simulink model "controller_sdfp_host"  (Simulink 7.8)
settings: Solver=ode3  StartTime=0.0  StopTime=1  RelTol=1e-3
values from neighbouring files (symbols this model uses):
  delay_shift1 = -k_preint    (= 0)    [one_bit_control.m]
  delay_shift2 = -k_preint    (= 0)    [one_bit_control.m]
  delay_shift3 = -k_preint    (= 0)    [one_bit_control.m]
  fixpt_adder_in_bitwidth = w    (= 24)    [one_bit_control.m]    (also in reconstruction_filter_setup.m)
  fixpt_adder_in_position = d    (= 16)    [one_bit_control.m]    (also in reconstruction_filter_setup.m)
  fixpt_adder_out_bitwidth = w    (= 24)    [one_bit_control.m]    (also in reconstruction_filter_setup.m)
  fixpt_adder_out_position = d    (= 16)    [one_bit_control.m]    (also in reconstruction_filter_setup.m)
  fixpt_gain_bitwidth = w    (= 24)    [one_bit_control.m]    (also in reconstruction_filter_setup.m)
  fixpt_gain_position = d    (= 16)    [one_bit_control.m]    (also in reconstruction_filter_setup.m)
  k = 2^k_bitshift    (= 0.000244140625)    [one_bit_control.m]
  p0 = 1326*T^3*k^-3    [one_bit_control.m]
  p1 = 9397*T^2*k^-2    [one_bit_control.m]
  p2 = 262.3*T*k^-1    [one_bit_control.m]
  p3 = 16.65    [one_bit_control.m]
  postint_gain1 = k_postint    (= -12)    [one_bit_control.m]
  postint_gain2 = k_postint    (= -12)    [one_bit_control.m]
  postint_gain3 = k_postint    (= -12)    [one_bit_control.m]
  preint_gain1 = k_preint    (= 0)    [one_bit_control.m]
  preint_gain2 = k_preint    (= 0)    [one_bit_control.m]
  preint_gain3 = k_preint    (= 0)    [one_bit_control.m]
  q0 = 0*T^3*k^-3    [one_bit_control.m]
  q1 = 400.8*T^2*k^-2    [one_bit_control.m]
  q2 = 33.2*T*k^-1    [one_bit_control.m]
  T = ts    [one_bit_control.m]
  ts = 1/Fs    [one_bit_control.m]
libraries: simulink x4, commnoisgen2 x1, cstblocks x1
(part 2 of 2)

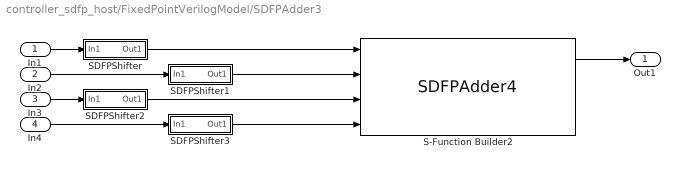
== system controller_sdfp_host/FixedPointVerilogModel/SDFPAdder3 ==
  In1 : Inport
  In2 : Inport  Port=2
  In3 : Inport  Port=3
  In4 : Inport  Port=4
  S-Function Builder2 : S-Function  InitFcn=try, set_param(gcb,'FunctionName','SDFPAdder4'), end  FunctionName=SDFPAdder4  Parameters=uint32(in_bitwidth),uint32(in_fp_position),uint32(out_bitwidth),uint32(out_fp_position)  SFunctionModules=SDFPAdder4_wrapper  WizardData=DataTag25  EnableBusSupport=off  mask(S-Function Builder){}
      mask help: The S-Function Builder block creates a wrapper C-MEX S-function from your supplied C code with multiple input ports, output ports, and a variable number of scalar, vector, or matrix parameters. The input and output ports can propagate Simulink built-in data types, fixed-point datatypes, complex, frame, 1-D, and 2-D signals. This block also supports discrete and continuous states of type real. You can optionally have the block generate a TLC file to be used with Real-Time Workshop for code generation.
      mask init: same as controller_sdfp_host/FixedPointVerilogModel/FloatForScope1/S-Function Builder
      settings: CopyFcn=set_param(gcbh,'LinkStatus','none')  PreSaveFcn=try, set_param(gcb,'FunctionName','SDFPAdder4'), end  OpenFcn=sfunctionwizard(gcbh)
      mask Display: plot(val(:,1),val(:,2)),disp(sys)port_label('input',1,'in0')port_label('input',2,'in1')port_label('input',3,'in2')port_label('input',4,'in3')port_label('output',1,'adder_out')port_label('output',2,'DBG_in01')port_label('output',3,'DBG_in012')
  SDFPShifter : Subsystem  mask{shift_amount=in1_shift}
      mask init:
      | if(shift_amount > 0)
      |     dispval=sprintf('<< %d',shift_amount);
      | else
      |     dispval=sprintf('>> %d',-shift_amount);
      | end
      mask Display: disp(dispval);
  SDFPShifter1 : Subsystem  mask{shift_amount=in2_shift}
      mask init:
      | if(shift_amount > 0)
      |     dispval=sprintf('<< %d',shift_amount);
      | else
      |     dispval=sprintf('>> %d',-shift_amount);
      | end
      mask Display: disp(dispval);
  SDFPShifter2 : Subsystem  mask{shift_amount=in3_shift}
      mask init:
      | if(shift_amount > 0)
      |     dispval=sprintf('<< %d',shift_amount);
      | else
      |     dispval=sprintf('>> %d',-shift_amount);
      | end
      mask Display: disp(dispval);
  SDFPShifter3 : Subsystem  mask{shift_amount=in4_shift}
      mask init:
      | if(shift_amount > 0)
      |     dispval=sprintf('<< %d',shift_amount);
      | else
      |     dispval=sprintf('>> %d',-shift_amount);
      | end
      mask Display: disp(dispval);
  Out1 : Outport
  wires:
  In1/1 -> SDFPShifter/1(In1)
  In2/1 -> SDFPShifter1/1(In1)
  In3/1 -> SDFPShifter2/1(In1)
  In4/1 -> SDFPShifter3/1(In1)
  S-Function Builder2/1 -> Out1/1
  SDFPShifter/1(Out1) -> S-Function Builder2/1
  SDFPShifter1/1(Out1) -> S-Function Builder2/2
  SDFPShifter2/1(Out1) -> S-Function Builder2/3
  SDFPShifter3/1(Out1) -> S-Function Builder2/4

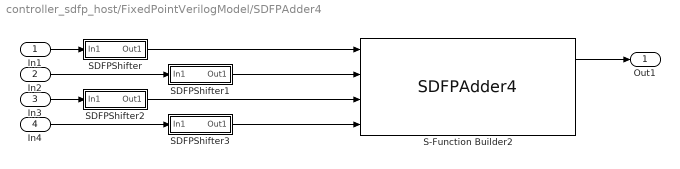
== system controller_sdfp_host/FixedPointVerilogModel/SDFPAdder4 ==
  In1 : Inport
  In2 : Inport  Port=2
  In3 : Inport  Port=3
  In4 : Inport  Port=4
  S-Function Builder2 : S-Function  InitFcn=try, set_param(gcb,'FunctionName','SDFPAdder4'), end  FunctionName=SDFPAdder4  Parameters=uint32(in_bitwidth),uint32(in_fp_position),uint32(out_bitwidth),uint32(out_fp_position)  SFunctionModules=SDFPAdder4_wrapper  WizardData=DataTag30  EnableBusSupport=off  mask(S-Function Builder){}
      mask help: The S-Function Builder block creates a wrapper C-MEX S-function from your supplied C code with multiple input ports, output ports, and a variable number of scalar, vector, or matrix parameters. The input and output ports can propagate Simulink built-in data types, fixed-point datatypes, complex, frame, 1-D, and 2-D signals. This block also supports discrete and continuous states of type real. You can optionally have the block generate a TLC file to be used with Real-Time Workshop for code generation.
      mask init: same as controller_sdfp_host/FixedPointVerilogModel/FloatForScope1/S-Function Builder
      settings: CopyFcn=set_param(gcbh,'LinkStatus','none')  PreSaveFcn=try, set_param(gcb,'FunctionName','SDFPAdder4'), end  OpenFcn=sfunctionwizard(gcbh)
      mask Display: plot(val(:,1),val(:,2)),disp(sys)port_label('input',1,'in0')port_label('input',2,'in1')port_label('input',3,'in2')port_label('input',4,'in3')port_label('output',1,'adder_out')port_label('output',2,'DBG_in01')port_label('output',3,'DBG_in012')
  SDFPShifter : Subsystem  mask{shift_amount=in1_shift}
      mask init:
      | if(shift_amount > 0)
      |     dispval=sprintf('<< %d',shift_amount);
      | else
      |     dispval=sprintf('>> %d',-shift_amount);
      | end
      mask Display: disp(dispval);
  SDFPShifter1 : Subsystem  mask{shift_amount=in2_shift}
      mask init:
      | if(shift_amount > 0)
      |     dispval=sprintf('<< %d',shift_amount);
      | else
      |     dispval=sprintf('>> %d',-shift_amount);
      | end
      mask Display: disp(dispval);
  SDFPShifter2 : Subsystem  mask{shift_amount=in3_shift}
      mask init:
      | if(shift_amount > 0)
      |     dispval=sprintf('<< %d',shift_amount);
      | else
      |     dispval=sprintf('>> %d',-shift_amount);
      | end
      mask Display: disp(dispval);
  SDFPShifter3 : Subsystem  mask{shift_amount=in4_shift}
      mask init:
      | if(shift_amount > 0)
      |     dispval=sprintf('<< %d',shift_amount);
      | else
      |     dispval=sprintf('>> %d',-shift_amount);
      | end
      mask Display: disp(dispval);
  Out1 : Outport
  wires:
  SDFPShifter3/1(Out1) -> S-Function Builder2/4
  SDFPShifter2/1(Out1) -> S-Function Builder2/3
  SDFPShifter1/1(Out1) -> S-Function Builder2/2
  SDFPShifter/1(Out1) -> S-Function Builder2/1
  S-Function Builder2/1 -> Out1/1
  In4/1 -> SDFPShifter3/1(In1)
  In3/1 -> SDFPShifter2/1(In1)
  In2/1 -> SDFPShifter1/1(In1)
  In1/1 -> SDFPShifter/1(In1)

== system controller_sdfp_host/FixedPointVerilogModel/ts_and_k_gain1 ==
  In1 : Inport
  S-Function Builder3 : S-Function  InitFcn=try, set_param(gcb,'FunctionName','SDFPShifter'), end  FunctionName=SDFPShifter  Parameters=int32(shift_amount)  SFunctionModules=SDFPShifter_wrapper  WizardData=DataTag35  EnableBusSupport=off  mask(S-Function Builder){}
      mask help: The S-Function Builder block creates a wrapper C-MEX S-function from your supplied C code with multiple input ports, output ports, and a variable number of scalar, vector, or matrix parameters. The input and output ports can propagate Simulink built-in data types, fixed-point datatypes, complex, frame, 1-D, and 2-D signals. This block also supports discrete and continuous states of type real. You can optionally have the block generate a TLC file to be used with Real-Time Workshop for code generation.
      mask init: same as controller_sdfp_host/FixedPointVerilogModel/FloatForScope1/S-Function Builder
      settings: CopyFcn=set_param(gcbh,'LinkStatus','none')  PreSaveFcn=try, set_param(gcb,'FunctionName','SDFPShifter'), end  OpenFcn=sfunctionwizard(gcbh)
      mask Display: plot(val(:,1),val(:,2)),disp(sys)port_label('input',1,'sg_in')port_label('output',1,'shifter_out')
  Out1 : Outport
  wires:
  In1/1 -> S-Function Builder3/1
  S-Function Builder3/1 -> Out1/1

== system controller_sdfp_host/FixedPointVerilogModel/ts_and_k_gain2 ==
  In1 : Inport
  S-Function Builder3 : S-Function  InitFcn=try, set_param(gcb,'FunctionName','SDFPShifter'), end  FunctionName=SDFPShifter  Parameters=int32(shift_amount)  SFunctionModules=SDFPShifter_wrapper  WizardData=DataTag36  EnableBusSupport=off  mask(S-Function Builder){}
      mask help: The S-Function Builder block creates a wrapper C-MEX S-function from your supplied C code with multiple input ports, output ports, and a variable number of scalar, vector, or matrix parameters. The input and output ports can propagate Simulink built-in data types, fixed-point datatypes, complex, frame, 1-D, and 2-D signals. This block also supports discrete and continuous states of type real. You can optionally have the block generate a TLC file to be used with Real-Time Workshop for code generation.
      mask init: same as controller_sdfp_host/FixedPointVerilogModel/FloatForScope1/S-Function Builder
      settings: CopyFcn=set_param(gcbh,'LinkStatus','none')  PreSaveFcn=try, set_param(gcb,'FunctionName','SDFPShifter'), end  OpenFcn=sfunctionwizard(gcbh)
      mask Display: plot(val(:,1),val(:,2)),disp(sys)port_label('input',1,'sg_in')port_label('output',1,'shifter_out')
  Out1 : Outport
  wires:
  S-Function Builder3/1 -> Out1/1
  In1/1 -> S-Function Builder3/1

== system controller_sdfp_host/FixedPointVerilogModel/ts_and_k_gain3 ==
  In1 : Inport
  S-Function Builder3 : S-Function  InitFcn=try, set_param(gcb,'FunctionName','SDFPShifter'), end  FunctionName=SDFPShifter  Parameters=int32(shift_amount)  SFunctionModules=SDFPShifter_wrapper  WizardData=DataTag37  EnableBusSupport=off  mask(S-Function Builder){}
      mask help: The S-Function Builder block creates a wrapper C-MEX S-function from your supplied C code with multiple input ports, output ports, and a variable number of scalar, vector, or matrix parameters. The input and output ports can propagate Simulink built-in data types, fixed-point datatypes, complex, frame, 1-D, and 2-D signals. This block also supports discrete and continuous states of type real. You can optionally have the block generate a TLC file to be used with Real-Time Workshop for code generation.
      mask init: same as controller_sdfp_host/FixedPointVerilogModel/FloatForScope1/S-Function Builder
      settings: CopyFcn=set_param(gcbh,'LinkStatus','none')  PreSaveFcn=try, set_param(gcb,'FunctionName','SDFPShifter'), end  OpenFcn=sfunctionwizard(gcbh)
      mask Display: plot(val(:,1),val(:,2)),disp(sys)port_label('input',1,'sg_in')port_label('output',1,'shifter_out')
  Out1 : Outport
  wires:
  In1/1 -> S-Function Builder3/1
  S-Function Builder3/1 -> Out1/1

== system controller_sdfp_host/FixedPointVerilogModel/ts_and_k_gain4 ==
  In1 : Inport
  S-Function Builder3 : S-Function  InitFcn=try, set_param(gcb,'FunctionName','SDFPShifter'), end  FunctionName=SDFPShifter  Parameters=int32(shift_amount)  SFunctionModules=SDFPShifter_wrapper  WizardData=DataTag38  EnableBusSupport=off  mask(S-Function Builder){}
      mask help: The S-Function Builder block creates a wrapper C-MEX S-function from your supplied C code with multiple input ports, output ports, and a variable number of scalar, vector, or matrix parameters. The input and output ports can propagate Simulink built-in data types, fixed-point datatypes, complex, frame, 1-D, and 2-D signals. This block also supports discrete and continuous states of type real. You can optionally have the block generate a TLC file to be used with Real-Time Workshop for code generation.
      mask init: same as controller_sdfp_host/FixedPointVerilogModel/FloatForScope1/S-Function Builder
      settings: CopyFcn=set_param(gcbh,'LinkStatus','none')  PreSaveFcn=try, set_param(gcb,'FunctionName','SDFPShifter'), end  OpenFcn=sfunctionwizard(gcbh)
      mask Display: plot(val(:,1),val(:,2)),disp(sys)port_label('input',1,'sg_in')port_label('output',1,'shifter_out')
  Out1 : Outport
  wires:
  In1/1 -> S-Function Builder3/1
  S-Function Builder3/1 -> Out1/1

== system controller_sdfp_host/FixedPointVerilogModel/ts_and_k_gain5 ==
  In1 : Inport
  S-Function Builder3 : S-Function  InitFcn=try, set_param(gcb,'FunctionName','SDFPShifter'), end  FunctionName=SDFPShifter  Parameters=int32(shift_amount)  SFunctionModules=SDFPShifter_wrapper  WizardData=DataTag39  EnableBusSupport=off  mask(S-Function Builder){}
      mask help: The S-Function Builder block creates a wrapper C-MEX S-function from your supplied C code with multiple input ports, output ports, and a variable number of scalar, vector, or matrix parameters. The input and output ports can propagate Simulink built-in data types, fixed-point datatypes, complex, frame, 1-D, and 2-D signals. This block also supports discrete and continuous states of type real. You can optionally have the block generate a TLC file to be used with Real-Time Workshop for code generation.
      mask init: same as controller_sdfp_host/FixedPointVerilogModel/FloatForScope1/S-Function Builder
      settings: CopyFcn=set_param(gcbh,'LinkStatus','none')  PreSaveFcn=try, set_param(gcb,'FunctionName','SDFPShifter'), end  OpenFcn=sfunctionwizard(gcbh)
      mask Display: plot(val(:,1),val(:,2)),disp(sys)port_label('input',1,'sg_in')port_label('output',1,'shifter_out')
  Out1 : Outport
  wires:
  In1/1 -> S-Function Builder3/1
  S-Function Builder3/1 -> Out1/1

== system controller_sdfp_host/FixedPointVerilogModel/ts_and_k_gain6 ==
  In1 : Inport
  S-Function Builder3 : S-Function  InitFcn=try, set_param(gcb,'FunctionName','SDFPShifter'), end  FunctionName=SDFPShifter  Parameters=int32(shift_amount)  SFunctionModules=SDFPShifter_wrapper  WizardData=DataTag40  EnableBusSupport=off  mask(S-Function Builder){}
      mask help: The S-Function Builder block creates a wrapper C-MEX S-function from your supplied C code with multiple input ports, output ports, and a variable number of scalar, vector, or matrix parameters. The input and output ports can propagate Simulink built-in data types, fixed-point datatypes, complex, frame, 1-D, and 2-D signals. This block also supports discrete and continuous states of type real. You can optionally have the block generate a TLC file to be used with Real-Time Workshop for code generation.
      mask init: same as controller_sdfp_host/FixedPointVerilogModel/FloatForScope1/S-Function Builder
      settings: CopyFcn=set_param(gcbh,'LinkStatus','none')  PreSaveFcn=try, set_param(gcb,'FunctionName','SDFPShifter'), end  OpenFcn=sfunctionwizard(gcbh)
      mask Display: plot(val(:,1),val(:,2)),disp(sys)port_label('input',1,'sg_in')port_label('output',1,'shifter_out')
  Out1 : Outport
  wires:
  S-Function Builder3/1 -> Out1/1
  In1/1 -> S-Function Builder3/1

== system controller_sdfp_host/SecondOrder Sigdel1/Compare to Zero ==
  In1 : Inport
  Compare To Zero : simulink/Logic and Bit Operations/Compare To Zero  relop=>=  OutDataTypeStr=uint8
  Constant : Constant
  Constant1 : Constant  Value=-1
  Switch : Switch  Threshold=0.5
  Out1 : Outport
  wires:
  Constant1/1 -> Switch/3
  Constant/1 -> Switch/1
  Compare To Zero/1 -> Switch/2
  In1/1 -> Compare To Zero/1
  Switch/1 -> Out1/1

== system controller_sdfp_host/SecondOrder Sigdel2/Compare to Zero ==
  In1 : Inport
  Compare To Zero : simulink/Logic and Bit Operations/Compare To Zero  relop=>=  OutDataTypeStr=uint8
  Constant : Constant
  Constant1 : Constant  Value=-1
  Switch : Switch  Threshold=0.5
  Out1 : Outport
  wires:
  Constant1/1 -> Switch/3
  Constant/1 -> Switch/1
  Compare To Zero/1 -> Switch/2
  In1/1 -> Compare To Zero/1
  Switch/1 -> Out1/1

== system controller_sdfp_host/SecondOrder Sigdel3/Compare to Zero ==
  In1 : Inport
  Compare To Zero : simulink/Logic and Bit Operations/Compare To Zero  relop=>=  OutDataTypeStr=uint8
  Constant : Constant
  Constant1 : Constant  Value=-1
  Switch : Switch  Threshold=0.5
  Out1 : Outport
  wires:
  Constant1/1 -> Switch/3
  Constant/1 -> Switch/1
  Compare To Zero/1 -> Switch/2
  In1/1 -> Compare To Zero/1
  Switch/1 -> Out1/1

== system controller_sdfp_host/FixedPointVerilogModel/SDFPAdder1/GM1Float ==
  In1 : Inport
  S-Function Builder : S-Function  InitFcn=try, set_param(gcb,'FunctionName','SDFPFromFixed'), end  FunctionName=SDFPFromFixed  Parameters=uint32(bitwidth),uint32(fp_position)  SFunctionModules=SDFPFromFixed_wrapper fpconv  WizardData=DataTag13  EnableBusSupport=off  mask(S-Function Builder){}
      mask help: The S-Function Builder block creates a wrapper C-MEX S-function from your supplied C code with multiple input ports, output ports, and a variable number of scalar, vector, or matrix parameters. The input and output ports can propagate Simulink built-in data types, fixed-point datatypes, complex, frame, 1-D, and 2-D signals. This block also supports discrete and continuous states of type real. You can optionally have the block generate a TLC file to be used with Real-Time Workshop for code generation.
      mask init: same as controller_sdfp_host/FixedPointVerilogModel/FloatForScope1/S-Function Builder
      settings: CopyFcn=set_param(gcbh,'LinkStatus','none')  PreSaveFcn=try, set_param(gcb,'FunctionName','SDFPFromFixed'), end  OpenFcn=sfunctionwizard(gcbh)
      mask Display: plot(val(:,1),val(:,2)),disp(sys)port_label('input',1,'fixed_in')port_label('output',1,'float_out')
  Out1 : Outport
  wires:
  In1/1 -> S-Function Builder/1
  S-Function Builder/1 -> Out1/1

== system controller_sdfp_host/FixedPointVerilogModel/SDFPAdder1/GM1Float1 ==
  In1 : Inport
  S-Function Builder : S-Function  InitFcn=try, set_param(gcb,'FunctionName','SDFPFromFixed'), end  FunctionName=SDFPFromFixed  Parameters=uint32(bitwidth),uint32(fp_position)  SFunctionModules=SDFPFromFixed_wrapper fpconv  WizardData=DataTag14  EnableBusSupport=off  mask(S-Function Builder){}
      mask help: The S-Function Builder block creates a wrapper C-MEX S-function from your supplied C code with multiple input ports, output ports, and a variable number of scalar, vector, or matrix parameters. The input and output ports can propagate Simulink built-in data types, fixed-point datatypes, complex, frame, 1-D, and 2-D signals. This block also supports discrete and continuous states of type real. You can optionally have the block generate a TLC file to be used with Real-Time Workshop for code generation.
      mask init: same as controller_sdfp_host/FixedPointVerilogModel/FloatForScope1/S-Function Builder
      settings: CopyFcn=set_param(gcbh,'LinkStatus','none')  PreSaveFcn=try, set_param(gcb,'FunctionName','SDFPFromFixed'), end  OpenFcn=sfunctionwizard(gcbh)
      mask Display: plot(val(:,1),val(:,2)),disp(sys)port_label('input',1,'fixed_in')port_label('output',1,'float_out')
  Out1 : Outport
  wires:
  In1/1 -> S-Function Builder/1
  S-Function Builder/1 -> Out1/1

== system controller_sdfp_host/FixedPointVerilogModel/SDFPAdder1/SDFPShifter ==
  In1 : Inport
  S-Function Builder3 : S-Function  InitFcn=try, set_param(gcb,'FunctionName','SDFPShifter'), end  FunctionName=SDFPShifter  Parameters=int32(shift_amount)  SFunctionModules=SDFPShifter_wrapper  WizardData=DataTag16  EnableBusSupport=off  mask(S-Function Builder){}
      mask help: The S-Function Builder block creates a wrapper C-MEX S-function from your supplied C code with multiple input ports, output ports, and a variable number of scalar, vector, or matrix parameters. The input and output ports can propagate Simulink built-in data types, fixed-point datatypes, complex, frame, 1-D, and 2-D signals. This block also supports discrete and continuous states of type real. You can optionally have the block generate a TLC file to be used with Real-Time Workshop for code generation.
      mask init: same as controller_sdfp_host/FixedPointVerilogModel/FloatForScope1/S-Function Builder
      settings: CopyFcn=set_param(gcbh,'LinkStatus','none')  PreSaveFcn=try, set_param(gcb,'FunctionName','SDFPShifter'), end  OpenFcn=sfunctionwizard(gcbh)
      mask Display: plot(val(:,1),val(:,2)),disp(sys)port_label('input',1,'sg_in')port_label('output',1,'shifter_out')
  Out1 : Outport
  wires:
  In1/1 -> S-Function Builder3/1
  S-Function Builder3/1 -> Out1/1

== system controller_sdfp_host/FixedPointVerilogModel/SDFPAdder1/SDFPShifter1 ==
  In1 : Inport
  S-Function Builder3 : S-Function  InitFcn=try, set_param(gcb,'FunctionName','SDFPShifter'), end  FunctionName=SDFPShifter  Parameters=int32(shift_amount)  SFunctionModules=SDFPShifter_wrapper  WizardData=DataTag17  EnableBusSupport=off  mask(S-Function Builder){}
      mask help: The S-Function Builder block creates a wrapper C-MEX S-function from your supplied C code with multiple input ports, output ports, and a variable number of scalar, vector, or matrix parameters. The input and output ports can propagate Simulink built-in data types, fixed-point datatypes, complex, frame, 1-D, and 2-D signals. This block also supports discrete and continuous states of type real. You can optionally have the block generate a TLC file to be used with Real-Time Workshop for code generation.
      mask init: same as controller_sdfp_host/FixedPointVerilogModel/FloatForScope1/S-Function Builder
      settings: CopyFcn=set_param(gcbh,'LinkStatus','none')  PreSaveFcn=try, set_param(gcb,'FunctionName','SDFPShifter'), end  OpenFcn=sfunctionwizard(gcbh)
      mask Display: plot(val(:,1),val(:,2)),disp(sys)port_label('input',1,'sg_in')port_label('output',1,'shifter_out')
  Out1 : Outport
  wires:
  S-Function Builder3/1 -> Out1/1
  In1/1 -> S-Function Builder3/1

== system controller_sdfp_host/FixedPointVerilogModel/SDFPAdder1/SDFPShifter2 ==
  In1 : Inport
  S-Function Builder3 : S-Function  InitFcn=try, set_param(gcb,'FunctionName','SDFPShifter'), end  FunctionName=SDFPShifter  Parameters=int32(shift_amount)  SFunctionModules=SDFPShifter_wrapper  WizardData=DataTag18  EnableBusSupport=off  mask(S-Function Builder){}
      mask help: The S-Function Builder block creates a wrapper C-MEX S-function from your supplied C code with multiple input ports, output ports, and a variable number of scalar, vector, or matrix parameters. The input and output ports can propagate Simulink built-in data types, fixed-point datatypes, complex, frame, 1-D, and 2-D signals. This block also supports discrete and continuous states of type real. You can optionally have the block generate a TLC file to be used with Real-Time Workshop for code generation.
      mask init: same as controller_sdfp_host/FixedPointVerilogModel/FloatForScope1/S-Function Builder
      settings: CopyFcn=set_param(gcbh,'LinkStatus','none')  PreSaveFcn=try, set_param(gcb,'FunctionName','SDFPShifter'), end  OpenFcn=sfunctionwizard(gcbh)
      mask Display: plot(val(:,1),val(:,2)),disp(sys)port_label('input',1,'sg_in')port_label('output',1,'shifter_out')
  Out1 : Outport
  wires:
  In1/1 -> S-Function Builder3/1
  S-Function Builder3/1 -> Out1/1

== system controller_sdfp_host/FixedPointVerilogModel/SDFPAdder1/SDFPShifter3 ==
  In1 : Inport
  S-Function Builder3 : S-Function  InitFcn=try, set_param(gcb,'FunctionName','SDFPShifter'), end  FunctionName=SDFPShifter  Parameters=int32(shift_amount)  SFunctionModules=SDFPShifter_wrapper  WizardData=DataTag19  EnableBusSupport=off  mask(S-Function Builder){}
      mask help: The S-Function Builder block creates a wrapper C-MEX S-function from your supplied C code with multiple input ports, output ports, and a variable number of scalar, vector, or matrix parameters. The input and output ports can propagate Simulink built-in data types, fixed-point datatypes, complex, frame, 1-D, and 2-D signals. This block also supports discrete and continuous states of type real. You can optionally have the block generate a TLC file to be used with Real-Time Workshop for code generation.
      mask init: same as controller_sdfp_host/FixedPointVerilogModel/FloatForScope1/S-Function Builder
      settings: CopyFcn=set_param(gcbh,'LinkStatus','none')  PreSaveFcn=try, set_param(gcb,'FunctionName','SDFPShifter'), end  OpenFcn=sfunctionwizard(gcbh)
      mask Display: plot(val(:,1),val(:,2)),disp(sys)port_label('input',1,'sg_in')port_label('output',1,'shifter_out')
  Out1 : Outport
  wires:
  S-Function Builder3/1 -> Out1/1
  In1/1 -> S-Function Builder3/1

== system controller_sdfp_host/FixedPointVerilogModel/SDFPAdder2/SDFPShifter ==
  In1 : Inport
  S-Function Builder3 : S-Function  InitFcn=try, set_param(gcb,'FunctionName','SDFPShifter'), end  FunctionName=SDFPShifter  Parameters=int32(shift_amount)  SFunctionModules=SDFPShifter_wrapper  WizardData=DataTag21  EnableBusSupport=off  mask(S-Function Builder){}
      mask help: The S-Function Builder block creates a wrapper C-MEX S-function from your supplied C code with multiple input ports, output ports, and a variable number of scalar, vector, or matrix parameters. The input and output ports can propagate Simulink built-in data types, fixed-point datatypes, complex, frame, 1-D, and 2-D signals. This block also supports discrete and continuous states of type real. You can optionally have the block generate a TLC file to be used with Real-Time Workshop for code generation.
      mask init: same as controller_sdfp_host/FixedPointVerilogModel/FloatForScope1/S-Function Builder
      settings: CopyFcn=set_param(gcbh,'LinkStatus','none')  PreSaveFcn=try, set_param(gcb,'FunctionName','SDFPShifter'), end  OpenFcn=sfunctionwizard(gcbh)
      mask Display: plot(val(:,1),val(:,2)),disp(sys)port_label('input',1,'sg_in')port_label('output',1,'shifter_out')
  Out1 : Outport
  wires:
  S-Function Builder3/1 -> Out1/1
  In1/1 -> S-Function Builder3/1

== system controller_sdfp_host/FixedPointVerilogModel/SDFPAdder2/SDFPShifter1 ==
  In1 : Inport
  S-Function Builder3 : S-Function  InitFcn=try, set_param(gcb,'FunctionName','SDFPShifter'), end  FunctionName=SDFPShifter  Parameters=int32(shift_amount)  SFunctionModules=SDFPShifter_wrapper  WizardData=DataTag22  EnableBusSupport=off  mask(S-Function Builder){}
      mask help: The S-Function Builder block creates a wrapper C-MEX S-function from your supplied C code with multiple input ports, output ports, and a variable number of scalar, vector, or matrix parameters. The input and output ports can propagate Simulink built-in data types, fixed-point datatypes, complex, frame, 1-D, and 2-D signals. This block also supports discrete and continuous states of type real. You can optionally have the block generate a TLC file to be used with Real-Time Workshop for code generation.
      mask init: same as controller_sdfp_host/FixedPointVerilogModel/FloatForScope1/S-Function Builder
      settings: CopyFcn=set_param(gcbh,'LinkStatus','none')  PreSaveFcn=try, set_param(gcb,'FunctionName','SDFPShifter'), end  OpenFcn=sfunctionwizard(gcbh)
      mask Display: plot(val(:,1),val(:,2)),disp(sys)port_label('input',1,'sg_in')port_label('output',1,'shifter_out')
  Out1 : Outport
  wires:
  In1/1 -> S-Function Builder3/1
  S-Function Builder3/1 -> Out1/1

== system controller_sdfp_host/FixedPointVerilogModel/SDFPAdder2/SDFPShifter2 ==
  In1 : Inport
  S-Function Builder3 : S-Function  InitFcn=try, set_param(gcb,'FunctionName','SDFPShifter'), end  FunctionName=SDFPShifter  Parameters=int32(shift_amount)  SFunctionModules=SDFPShifter_wrapper  WizardData=DataTag23  EnableBusSupport=off  mask(S-Function Builder){}
      mask help: The S-Function Builder block creates a wrapper C-MEX S-function from your supplied C code with multiple input ports, output ports, and a variable number of scalar, vector, or matrix parameters. The input and output ports can propagate Simulink built-in data types, fixed-point datatypes, complex, frame, 1-D, and 2-D signals. This block also supports discrete and continuous states of type real. You can optionally have the block generate a TLC file to be used with Real-Time Workshop for code generation.
      mask init: same as controller_sdfp_host/FixedPointVerilogModel/FloatForScope1/S-Function Builder
      settings: CopyFcn=set_param(gcbh,'LinkStatus','none')  PreSaveFcn=try, set_param(gcb,'FunctionName','SDFPShifter'), end  OpenFcn=sfunctionwizard(gcbh)
      mask Display: plot(val(:,1),val(:,2)),disp(sys)port_label('input',1,'sg_in')port_label('output',1,'shifter_out')
  Out1 : Outport
  wires:
  S-Function Builder3/1 -> Out1/1
  In1/1 -> S-Function Builder3/1

== system controller_sdfp_host/FixedPointVerilogModel/SDFPAdder2/SDFPShifter3 ==
  In1 : Inport
  S-Function Builder3 : S-Function  InitFcn=try, set_param(gcb,'FunctionName','SDFPShifter'), end  FunctionName=SDFPShifter  Parameters=int32(shift_amount)  SFunctionModules=SDFPShifter_wrapper  WizardData=DataTag24  EnableBusSupport=off  mask(S-Function Builder){}
      mask help: The S-Function Builder block creates a wrapper C-MEX S-function from your supplied C code with multiple input ports, output ports, and a variable number of scalar, vector, or matrix parameters. The input and output ports can propagate Simulink built-in data types, fixed-point datatypes, complex, frame, 1-D, and 2-D signals. This block also supports discrete and continuous states of type real. You can optionally have the block generate a TLC file to be used with Real-Time Workshop for code generation.
      mask init: same as controller_sdfp_host/FixedPointVerilogModel/FloatForScope1/S-Function Builder
      settings: CopyFcn=set_param(gcbh,'LinkStatus','none')  PreSaveFcn=try, set_param(gcb,'FunctionName','SDFPShifter'), end  OpenFcn=sfunctionwizard(gcbh)
      mask Display: plot(val(:,1),val(:,2)),disp(sys)port_label('input',1,'sg_in')port_label('output',1,'shifter_out')
  Out1 : Outport
  wires:
  In1/1 -> S-Function Builder3/1
  S-Function Builder3/1 -> Out1/1

== system controller_sdfp_host/FixedPointVerilogModel/SDFPAdder3/SDFPShifter ==
  In1 : Inport
  S-Function Builder3 : S-Function  InitFcn=try, set_param(gcb,'FunctionName','SDFPShifter'), end  FunctionName=SDFPShifter  Parameters=int32(shift_amount)  SFunctionModules=SDFPShifter_wrapper  WizardData=DataTag26  EnableBusSupport=off  mask(S-Function Builder){}
      mask help: The S-Function Builder block creates a wrapper C-MEX S-function from your supplied C code with multiple input ports, output ports, and a variable number of scalar, vector, or matrix parameters. The input and output ports can propagate Simulink built-in data types, fixed-point datatypes, complex, frame, 1-D, and 2-D signals. This block also supports discrete and continuous states of type real. You can optionally have the block generate a TLC file to be used with Real-Time Workshop for code generation.
      mask init: same as controller_sdfp_host/FixedPointVerilogModel/FloatForScope1/S-Function Builder
      settings: CopyFcn=set_param(gcbh,'LinkStatus','none')  PreSaveFcn=try, set_param(gcb,'FunctionName','SDFPShifter'), end  OpenFcn=sfunctionwizard(gcbh)
      mask Display: plot(val(:,1),val(:,2)),disp(sys)port_label('input',1,'sg_in')port_label('output',1,'shifter_out')
  Out1 : Outport
  wires:
  In1/1 -> S-Function Builder3/1
  S-Function Builder3/1 -> Out1/1

== system controller_sdfp_host/FixedPointVerilogModel/SDFPAdder3/SDFPShifter1 ==
  In1 : Inport
  S-Function Builder3 : S-Function  InitFcn=try, set_param(gcb,'FunctionName','SDFPShifter'), end  FunctionName=SDFPShifter  Parameters=int32(shift_amount)  SFunctionModules=SDFPShifter_wrapper  WizardData=DataTag27  EnableBusSupport=off  mask(S-Function Builder){}
      mask help: The S-Function Builder block creates a wrapper C-MEX S-function from your supplied C code with multiple input ports, output ports, and a variable number of scalar, vector, or matrix parameters. The input and output ports can propagate Simulink built-in data types, fixed-point datatypes, complex, frame, 1-D, and 2-D signals. This block also supports discrete and continuous states of type real. You can optionally have the block generate a TLC file to be used with Real-Time Workshop for code generation.
      mask init: same as controller_sdfp_host/FixedPointVerilogModel/FloatForScope1/S-Function Builder
      settings: CopyFcn=set_param(gcbh,'LinkStatus','none')  PreSaveFcn=try, set_param(gcb,'FunctionName','SDFPShifter'), end  OpenFcn=sfunctionwizard(gcbh)
      mask Display: plot(val(:,1),val(:,2)),disp(sys)port_label('input',1,'sg_in')port_label('output',1,'shifter_out')
  Out1 : Outport
  wires:
  S-Function Builder3/1 -> Out1/1
  In1/1 -> S-Function Builder3/1

== system controller_sdfp_host/FixedPointVerilogModel/SDFPAdder3/SDFPShifter2 ==
  In1 : Inport
  S-Function Builder3 : S-Function  InitFcn=try, set_param(gcb,'FunctionName','SDFPShifter'), end  FunctionName=SDFPShifter  Parameters=int32(shift_amount)  SFunctionModules=SDFPShifter_wrapper  WizardData=DataTag28  EnableBusSupport=off  mask(S-Function Builder){}
      mask help: The S-Function Builder block creates a wrapper C-MEX S-function from your supplied C code with multiple input ports, output ports, and a variable number of scalar, vector, or matrix parameters. The input and output ports can propagate Simulink built-in data types, fixed-point datatypes, complex, frame, 1-D, and 2-D signals. This block also supports discrete and continuous states of type real. You can optionally have the block generate a TLC file to be used with Real-Time Workshop for code generation.
      mask init: same as controller_sdfp_host/FixedPointVerilogModel/FloatForScope1/S-Function Builder
      settings: CopyFcn=set_param(gcbh,'LinkStatus','none')  PreSaveFcn=try, set_param(gcb,'FunctionName','SDFPShifter'), end  OpenFcn=sfunctionwizard(gcbh)
      mask Display: plot(val(:,1),val(:,2)),disp(sys)port_label('input',1,'sg_in')port_label('output',1,'shifter_out')
  Out1 : Outport
  wires:
  In1/1 -> S-Function Builder3/1
  S-Function Builder3/1 -> Out1/1

== system controller_sdfp_host/FixedPointVerilogModel/SDFPAdder3/SDFPShifter3 ==
  In1 : Inport
  S-Function Builder3 : S-Function  InitFcn=try, set_param(gcb,'FunctionName','SDFPShifter'), end  FunctionName=SDFPShifter  Parameters=int32(shift_amount)  SFunctionModules=SDFPShifter_wrapper  WizardData=DataTag29  EnableBusSupport=off  mask(S-Function Builder){}
      mask help: The S-Function Builder block creates a wrapper C-MEX S-function from your supplied C code with multiple input ports, output ports, and a variable number of scalar, vector, or matrix parameters. The input and output ports can propagate Simulink built-in data types, fixed-point datatypes, complex, frame, 1-D, and 2-D signals. This block also supports discrete and continuous states of type real. You can optionally have the block generate a TLC file to be used with Real-Time Workshop for code generation.
      mask init: same as controller_sdfp_host/FixedPointVerilogModel/FloatForScope1/S-Function Builder
      settings: CopyFcn=set_param(gcbh,'LinkStatus','none')  PreSaveFcn=try, set_param(gcb,'FunctionName','SDFPShifter'), end  OpenFcn=sfunctionwizard(gcbh)
      mask Display: plot(val(:,1),val(:,2)),disp(sys)port_label('input',1,'sg_in')port_label('output',1,'shifter_out')
  Out1 : Outport
  wires:
  S-Function Builder3/1 -> Out1/1
  In1/1 -> S-Function Builder3/1

== system controller_sdfp_host/FixedPointVerilogModel/SDFPAdder4/SDFPShifter ==
  In1 : Inport
  S-Function Builder3 : S-Function  InitFcn=try, set_param(gcb,'FunctionName','SDFPShifter'), end  FunctionName=SDFPShifter  Parameters=int32(shift_amount)  SFunctionModules=SDFPShifter_wrapper  WizardData=DataTag31  EnableBusSupport=off  mask(S-Function Builder){}
      mask help: The S-Function Builder block creates a wrapper C-MEX S-function from your supplied C code with multiple input ports, output ports, and a variable number of scalar, vector, or matrix parameters. The input and output ports can propagate Simulink built-in data types, fixed-point datatypes, complex, frame, 1-D, and 2-D signals. This block also supports discrete and continuous states of type real. You can optionally have the block generate a TLC file to be used with Real-Time Workshop for code generation.
      mask init: same as controller_sdfp_host/FixedPointVerilogModel/FloatForScope1/S-Function Builder
      settings: CopyFcn=set_param(gcbh,'LinkStatus','none')  PreSaveFcn=try, set_param(gcb,'FunctionName','SDFPShifter'), end  OpenFcn=sfunctionwizard(gcbh)
      mask Display: plot(val(:,1),val(:,2)),disp(sys)port_label('input',1,'sg_in')port_label('output',1,'shifter_out')
  Out1 : Outport
  wires:
  S-Function Builder3/1 -> Out1/1
  In1/1 -> S-Function Builder3/1

== system controller_sdfp_host/FixedPointVerilogModel/SDFPAdder4/SDFPShifter1 ==
  In1 : Inport
  S-Function Builder3 : S-Function  InitFcn=try, set_param(gcb,'FunctionName','SDFPShifter'), end  FunctionName=SDFPShifter  Parameters=int32(shift_amount)  SFunctionModules=SDFPShifter_wrapper  WizardData=DataTag32  EnableBusSupport=off  mask(S-Function Builder){}
      mask help: The S-Function Builder block creates a wrapper C-MEX S-function from your supplied C code with multiple input ports, output ports, and a variable number of scalar, vector, or matrix parameters. The input and output ports can propagate Simulink built-in data types, fixed-point datatypes, complex, frame, 1-D, and 2-D signals. This block also supports discrete and continuous states of type real. You can optionally have the block generate a TLC file to be used with Real-Time Workshop for code generation.
      mask init: same as controller_sdfp_host/FixedPointVerilogModel/FloatForScope1/S-Function Builder
      settings: CopyFcn=set_param(gcbh,'LinkStatus','none')  PreSaveFcn=try, set_param(gcb,'FunctionName','SDFPShifter'), end  OpenFcn=sfunctionwizard(gcbh)
      mask Display: plot(val(:,1),val(:,2)),disp(sys)port_label('input',1,'sg_in')port_label('output',1,'shifter_out')
  Out1 : Outport
  wires:
  In1/1 -> S-Function Builder3/1
  S-Function Builder3/1 -> Out1/1

== system controller_sdfp_host/FixedPointVerilogModel/SDFPAdder4/SDFPShifter2 ==
  In1 : Inport
  S-Function Builder3 : S-Function  InitFcn=try, set_param(gcb,'FunctionName','SDFPShifter'), end  FunctionName=SDFPShifter  Parameters=int32(shift_amount)  SFunctionModules=SDFPShifter_wrapper  WizardData=DataTag33  EnableBusSupport=off  mask(S-Function Builder){}
      mask help: The S-Function Builder block creates a wrapper C-MEX S-function from your supplied C code with multiple input ports, output ports, and a variable number of scalar, vector, or matrix parameters. The input and output ports can propagate Simulink built-in data types, fixed-point datatypes, complex, frame, 1-D, and 2-D signals. This block also supports discrete and continuous states of type real. You can optionally have the block generate a TLC file to be used with Real-Time Workshop for code generation.
      mask init: same as controller_sdfp_host/FixedPointVerilogModel/FloatForScope1/S-Function Builder
      settings: CopyFcn=set_param(gcbh,'LinkStatus','none')  PreSaveFcn=try, set_param(gcb,'FunctionName','SDFPShifter'), end  OpenFcn=sfunctionwizard(gcbh)
      mask Display: plot(val(:,1),val(:,2)),disp(sys)port_label('input',1,'sg_in')port_label('output',1,'shifter_out')
  Out1 : Outport
  wires:
  S-Function Builder3/1 -> Out1/1
  In1/1 -> S-Function Builder3/1

== system controller_sdfp_host/FixedPointVerilogModel/SDFPAdder4/SDFPShifter3 ==
  In1 : Inport
  S-Function Builder3 : S-Function  InitFcn=try, set_param(gcb,'FunctionName','SDFPShifter'), end  FunctionName=SDFPShifter  Parameters=int32(shift_amount)  SFunctionModules=SDFPShifter_wrapper  WizardData=DataTag34  EnableBusSupport=off  mask(S-Function Builder){}
      mask help: The S-Function Builder block creates a wrapper C-MEX S-function from your supplied C code with multiple input ports, output ports, and a variable number of scalar, vector, or matrix parameters. The input and output ports can propagate Simulink built-in data types, fixed-point datatypes, complex, frame, 1-D, and 2-D signals. This block also supports discrete and continuous states of type real. You can optionally have the block generate a TLC file to be used with Real-Time Workshop for code generation.
      mask init: same as controller_sdfp_host/FixedPointVerilogModel/FloatForScope1/S-Function Builder
      settings: CopyFcn=set_param(gcbh,'LinkStatus','none')  PreSaveFcn=try, set_param(gcb,'FunctionName','SDFPShifter'), end  OpenFcn=sfunctionwizard(gcbh)
      mask Display: plot(val(:,1),val(:,2)),disp(sys)port_label('input',1,'sg_in')port_label('output',1,'shifter_out')
  Out1 : Outport
  wires:
  In1/1 -> S-Function Builder3/1
  S-Function Builder3/1 -> Out1/1
